simulink model "DeMultiplexer1x4"  (R2025b)
settings: Solver=VariableStepAuto  StartTime=0.0  StopTime=10.0  RelTol=1e-3
settings Model: Creator=jerin  LastModifiedBy=Johan

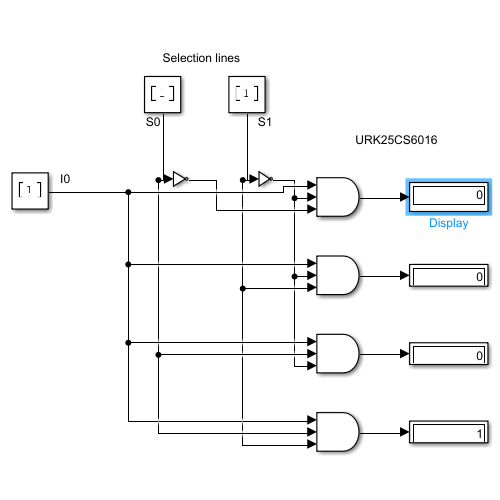
[thumbnail: Simulink's stored preview of the top-level diagram]
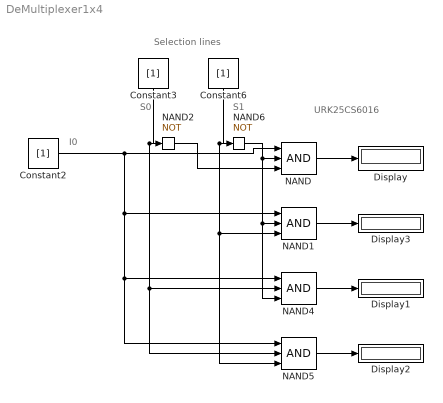
== system DeMultiplexer1x4 ==
  note: S1
  note: S0
  note: Selection lines
  note: I0
  note: URK25CS6016
  Constant2 : Constant  Value=[1]
  Constant3 : Constant  Value=[1]
  Constant6 : Constant  Value=[1]
  Display{,1..3} (4 alike) : Display
  NAND{,1,4..5} (4 alike) : Logic  Inputs=3  IconShape=distinctive  AllPortsSameDT=off  OutDataTypeStr=boolean
  NAND2 : Logic  Operator=NOT  IconShape=distinctive  AllPortsSameDT=off  OutDataTypeStr=boolean
  NAND6 : Logic  Operator=NOT  IconShape=distinctive  AllPortsSameDT=off  OutDataTypeStr=boolean
  wires:
  Constant2/1 -> NAND5/1, NAND4/1, NAND1/1, NAND/1
  Constant6/1 -> NAND5/3, NAND1/3, NAND6/1
  Constant3/1 -> NAND5/2, NAND4/2, NAND2/1
  NAND2/1 -> NAND/3
  NAND6/1 -> NAND4/3, NAND1/2, NAND/2
  NAND/1 -> Display/1
  NAND1/1 -> Display3/1
  NAND4/1 -> Display1/1
  NAND5/1 -> Display2/1
